simulink subsystem "State2Pose"  (R2023b)
settings: Solver=VariableStepAuto  StartTime=0.0  StopTime=10.0  RelTol=1e-3
undefined symbols (not defined in the file): ActorID, AngularVelocity, EgoCar1_params, Pitch, Position, Roll, Velocity, Yaw
settings Model: Creator=victor  LastModifiedBy=victor

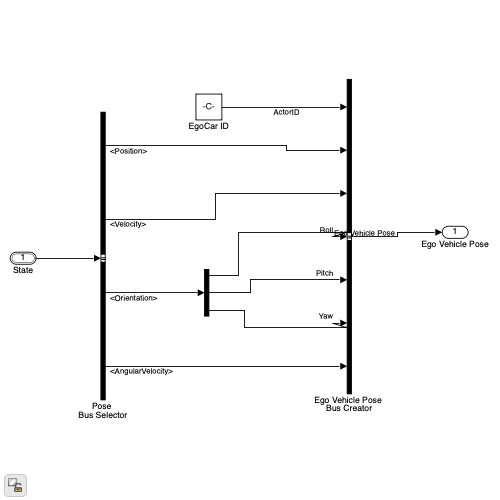
[thumbnail: Simulink's stored preview of the top-level diagram]
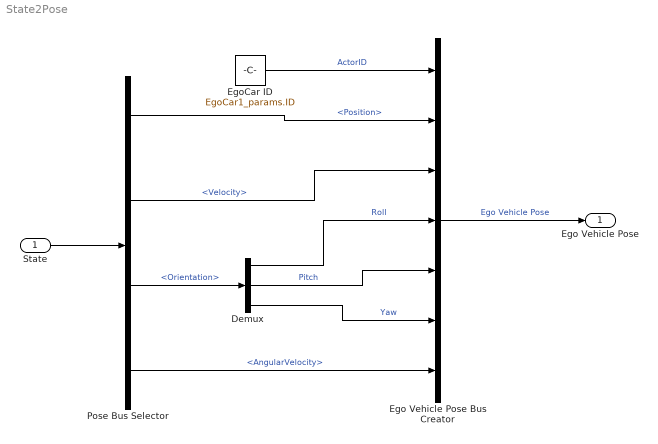
== system State2Pose ==
  State : Inport  OutDataTypeStr=Bus: BusEgoVehicleState
  Demux : Demux  Outputs=3
  Ego Vehicle Pose Bus Creator : BusCreator  Inputs=ActorID,Position,Velocity,Roll,Pitch,Yaw,AngularVelocity  OutDataTypeStr=Bus: BusEgoVehiclePose  NonVirtualBus=on
  EgoCar ID : Constant  Value=EgoCar1_params.ID
  Pose Bus Selector : BusSelector  OutputSignals=Position,Velocity,Orientation,AngularVelocity
  Ego Vehicle Pose : Outport  OutDataTypeStr=Bus: BusEgoVehiclePose
  wires:
  Pose Bus Selector/3 -> Demux/1  "<Orientation>"
  State/1 -> Pose Bus Selector/1
  Demux/1 -> Ego Vehicle Pose Bus Creator/4  "Roll"
  Demux/2 -> Ego Vehicle Pose Bus Creator/5  "Pitch"
  Demux/3 -> Ego Vehicle Pose Bus Creator/6  "Yaw"
  Ego Vehicle Pose Bus Creator/1 -> Ego Vehicle Pose/1  "Ego Vehicle Pose"
  Pose Bus Selector/1 -> Ego Vehicle Pose Bus Creator/2  "<Position>"
  Pose Bus Selector/2 -> Ego Vehicle Pose Bus Creator/3  "<Velocity>"
  Pose Bus Selector/4 -> Ego Vehicle Pose Bus Creator/7  "<AngularVelocity>"
  EgoCar ID/1 -> Ego Vehicle Pose Bus Creator/1  "ActorID"
